simulink model "MyModel_Open_v1"  (R2018b)
settings: Solver=VariableStepAuto  StartTime=0.0  StopTime=10.0  RelTol=1e-3
InitFcn:
  | Udc1 = 100;
  | Udc2 = 100;
undefined symbols (not defined in the file): tpwm
libraries: powerlib x31, powerlib_meascontrol x28, powerlib_extras x5, simulink x2
(part 1 of 2)
settings Model: Creator=chenhao  LastModifiedBy=chenhao

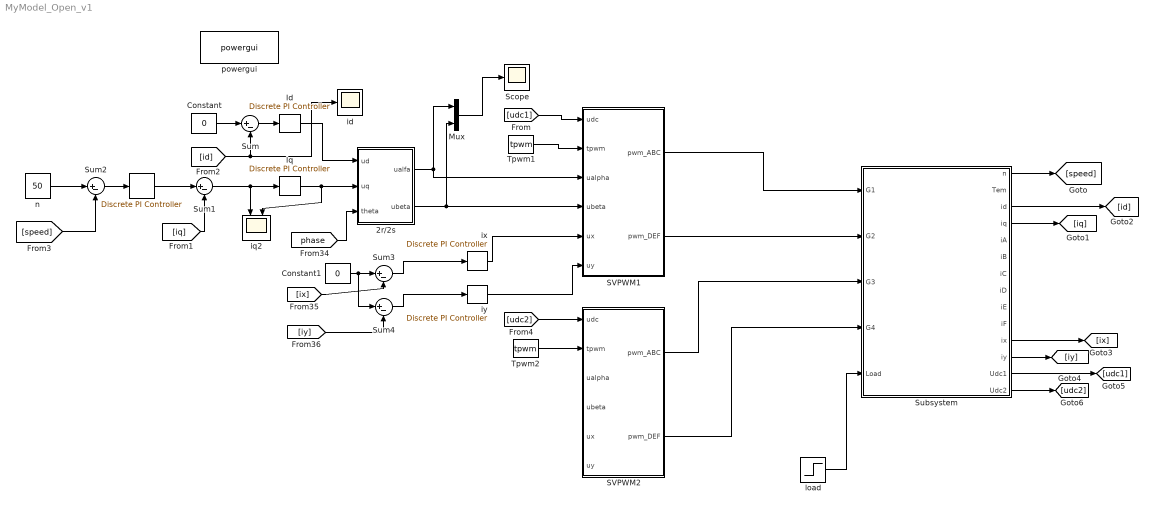
== system MyModel_Open_v1 ==
  "    " : powerlib_extras/Discrete  Control Blocks/Discrete PI Controller  Kp=1  Ki=80  Par_Limits=[50 -50]  Init=0  Ts=tpwm
  " Id" : powerlib_extras/Discrete  Control Blocks/Discrete PI Controller  Kp=3  Ki=120  Par_Limits=[300 -300]  Init=0  Ts=tpwm
  " Iq" : powerlib_extras/Discrete  Control Blocks/Discrete PI Controller  Kp=3  Ki=120  Par_Limits=[300 -300]  Init=0  Ts=tpwm
  " ix" : powerlib_extras/Discrete  Control Blocks/Discrete PI Controller  Kp=10  Ki=100  Par_Limits=[300 -300]  Init=0  Ts=tpwm
  " iy" : powerlib_extras/Discrete  Control Blocks/Discrete PI Controller  Kp=10  Ki=100  Par_Limits=[300 -300]  Init=0  Ts=tpwm
  2r/2s : Subsystem
  Constant : Constant  Value=0
  Constant1 : Constant  Value=0
  Mux : Mux  Inputs=2
  SVPWM1 : Subsystem
  SVPWM2 : Subsystem
  Scope : Scope
  Subsystem : Subsystem
  Sum{,1..4} (5 alike) : Sum  Inputs=|+-
  Tpwm1 : Constant  Value=tpwm
  Tpwm2 : Constant  Value=tpwm
  "id " : Scope
  iq2 : Scope  NumInputPorts=2
  load : Step  Time=0  After=15  SampleTime=0
  n : Constant  Value=50
  powergui : powerlib/powergui  Priority=1  SimulationMode=Discrete  SampleTime=5e-7  frequency=60  Iterations=50  frequencyindice=0  Pbase=100e6  ErrMax=1e-4  UnitsV=kV  UnitsW=MW  buscounter=0  FunctionMessages=off  echomessages=off  EnableUseOfTLC=off  CurrentSourceSwitches=off  DisableSnubberDevices=off  DisableRonSwitches=off  DisableVfSwitches=off  DisplayEquations=off  SolverType=Tustin  Interpol=off  ExternalGateDelay=off  methode=off  Ts=0  x0status=blocks  SPID=off  SwTol=0  HookPort=off  RestoreLinks=warning  ResistiveCurrentMeasurement=off  Frange=[0:2:500]  Ylog=off  Xlog=on  ShowGrid=off  save=off  variable=ZData  structure=Ia  ZoomFFT=on  StartTime=0.1  cycles=2  DisplayStyle=1  fundamental=2.5  FreqAxis=on  MaxFrequency=30  frequencyindicesteady=1  RmsSteady=1  display=off
  wires:
  2r/2s/2(ubeta) -> Mux/2, SVPWM1/4(ubeta)
  " ix"/1 -> SVPWM1/5(ux)
  Mux/1 -> Scope/1
  Tpwm1/1 -> SVPWM1/2(tpwm)
  load/1 -> Subsystem/5(Load)
  [iy] -> Sum4/2
  [iq] -> Sum1/2
  Sum3/1 -> " ix"/1
  [udc1] -> SVPWM1/1(udc)
  SVPWM1/1(pwm_ABC) -> Subsystem/1(G1)
  SVPWM1/2(pwm_DEF) -> Subsystem/2(G2)
  Sum2/1 -> "    "/1
  2r/2s/1(ualfa) -> Mux/1, SVPWM1/3(ualpha)
  Sum1/1 -> iq2/1, " Iq"/1
  [speed] -> Sum2/2
  Sum4/1 -> " iy"/1
  n/1 -> Sum2/1
  [ix] -> Sum3/2
  " Id"/1 -> 2r/2s/1(ud)
  [phase] -> 2r/2s/3(theta)
  " Iq"/1 -> iq2/2, 2r/2s/2(uq)
  Sum/1 -> " Id"/1
  Constant1/1 -> Sum4/1, Sum3/1
  "    "/1 -> Sum1/1
  " iy"/1 -> SVPWM1/6(uy)
  [id] -> "id "/1, Sum/2
  Constant/1 -> Sum/1
  Subsystem/1(n) -> [speed]
  Subsystem/4(iq) -> [iq]
  Subsystem/3(id) -> [id]
  Subsystem/11(ix) -> [ix]
  Subsystem/12(iy) -> [iy]
  Subsystem/13(Udc1) -> [udc1]
  Subsystem/14(Udc2) -> [udc2]
  [udc2] -> SVPWM2/1(udc)
  Tpwm2/1 -> SVPWM2/2(tpwm)
  SVPWM2/1(pwm_ABC) -> Subsystem/3(G3)
  SVPWM2/2(pwm_DEF) -> Subsystem/4(G4)

== system MyModel_Open_v1/2r//2s ==
  ud : Inport
  uq : Inport  Port=2
  theta : Inport  Port=3
  Fcn : Fcn  Expr=u(1)*cos(u(3))-u(2)*sin(u(3))
  Fcn1 : Fcn  Expr=u(1)*sin(u(3))+u(2)*cos(u(3))
  Mux1 : Mux  Inputs=3
  ualfa : Outport
  ubeta : Outport  Port=2
  wires:
  theta/1 -> Mux1/3
  uq/1 -> Mux1/2
  ud/1 -> Mux1/1
  Fcn1/1 -> ubeta/1
  Fcn/1 -> ualfa/1
  Mux1/1 -> Fcn1/1, Fcn/1

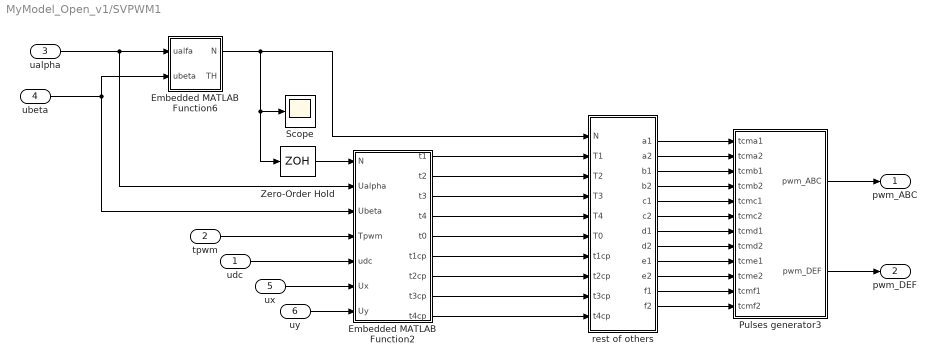
== system MyModel_Open_v1/SVPWM1 ==
  udc : Inport
  tpwm : Inport  Port=2
  ualpha : Inport  Port=3
  ubeta : Inport  Port=4
  ux : Inport  Port=5
  uy : Inport  Port=6
  Embedded MATLAB Function2 : MATLAB Function  TreatAsAtomicUnit=on
  Embedded MATLAB Function6 : MATLAB Function  TreatAsAtomicUnit=on
  Pulses generator3 : Subsystem
  Scope : Scope
  Zero-Order Hold : ZeroOrderHold  SampleTime=1e-4
  rest of others : MATLAB Function  TreatAsAtomicUnit=on
  pwm_ABC : Outport
  pwm_DEF : Outport  Port=2
  wires:
  udc/1 -> Embedded MATLAB Function2/5(udc)
  Embedded MATLAB Function2/4(t4) -> rest of others/5(T4)
  Embedded MATLAB Function2/1(t1) -> rest of others/2(T1)
  Pulses generator3/1(pwm_ABC) -> pwm_ABC/1
  Pulses generator3/2(pwm_DEF) -> pwm_DEF/1
  rest of others/12(f2) -> Pulses generator3/12(tcmf2)
  rest of others/11(f1) -> Pulses generator3/11(tcmf1)
  rest of others/10(e2) -> Pulses generator3/10(tcme2)
  rest of others/9(e1) -> Pulses generator3/9(tcme1)
  rest of others/8(d2) -> Pulses generator3/8(tcmd2)
  rest of others/7(d1) -> Pulses generator3/7(tcmd1)
  rest of others/6(c2) -> Pulses generator3/6(tcmc2)
  rest of others/5(c1) -> Pulses generator3/5(tcmc1)
  rest of others/4(b2) -> Pulses generator3/4(tcmb2)
  rest of others/3(b1) -> Pulses generator3/3(tcmb1)
  rest of others/2(a2) -> Pulses generator3/2(tcma2)
  rest of others/1(a1) -> Pulses generator3/1(tcma1)
  Embedded MATLAB Function2/2(t2) -> rest of others/3(T2)
  tpwm/1 -> Embedded MATLAB Function2/4(Tpwm)
  Embedded MATLAB Function2/5(t0) -> rest of others/6(T0)
  ualpha/1 -> Embedded MATLAB Function2/2(Ualpha), Embedded MATLAB Function6/1(ualfa)
  ubeta/1 -> Embedded MATLAB Function6/2(ubeta), Embedded MATLAB Function2/3(Ubeta)
  ux/1 -> Embedded MATLAB Function2/6(Ux)
  uy/1 -> Embedded MATLAB Function2/7(Uy)
  Embedded MATLAB Function2/3(t3) -> rest of others/4(T3)
  Zero-Order Hold/1 -> Embedded MATLAB Function2/1(N)
  Embedded MATLAB Function6/1(N) -> rest of others/1(N), Scope/1, Zero-Order Hold/1
  Embedded MATLAB Function2/9(t4cp) -> rest of others/10(t4cp)
  Embedded MATLAB Function2/8(t3cp) -> rest of others/9(t3cp)
  Embedded MATLAB Function2/7(t2cp) -> rest of others/8(t2cp)
  Embedded MATLAB Function2/6(t1cp) -> rest of others/7(t1cp)

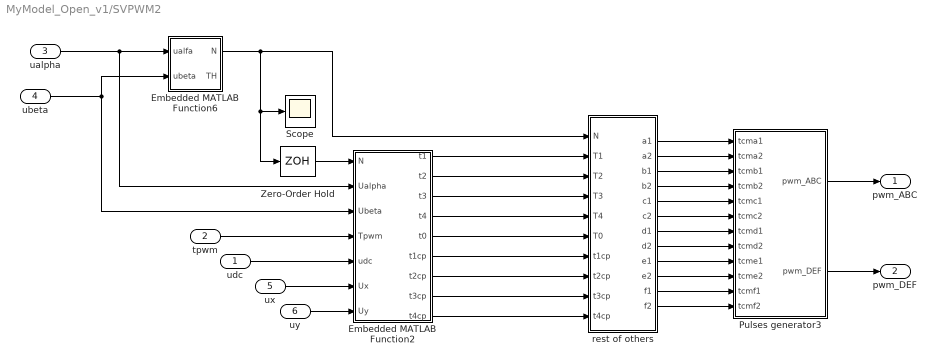
== system MyModel_Open_v1/SVPWM2 ==
  udc : Inport
  tpwm : Inport  Port=2
  ualpha : Inport  Port=3
  ubeta : Inport  Port=4
  ux : Inport  Port=5
  uy : Inport  Port=6
  Embedded MATLAB Function2 : MATLAB Function  TreatAsAtomicUnit=on
  Embedded MATLAB Function6 : MATLAB Function  TreatAsAtomicUnit=on
  Pulses generator3 : Subsystem
  Scope : Scope
  Zero-Order Hold : ZeroOrderHold  SampleTime=1e-4
  rest of others : MATLAB Function  TreatAsAtomicUnit=on
  pwm_ABC : Outport
  pwm_DEF : Outport  Port=2
  wires:
  Embedded MATLAB Function2/6(t1cp) -> rest of others/7(t1cp)
  Embedded MATLAB Function2/7(t2cp) -> rest of others/8(t2cp)
  Embedded MATLAB Function2/8(t3cp) -> rest of others/9(t3cp)
  Embedded MATLAB Function2/9(t4cp) -> rest of others/10(t4cp)
  Embedded MATLAB Function6/1(N) -> Zero-Order Hold/1, Scope/1, rest of others/1(N)
  Zero-Order Hold/1 -> Embedded MATLAB Function2/1(N)
  Embedded MATLAB Function2/3(t3) -> rest of others/4(T3)
  uy/1 -> Embedded MATLAB Function2/7(Uy)
  ux/1 -> Embedded MATLAB Function2/6(Ux)
  ubeta/1 -> Embedded MATLAB Function2/3(Ubeta), Embedded MATLAB Function6/2(ubeta)
  ualpha/1 -> Embedded MATLAB Function6/1(ualfa), Embedded MATLAB Function2/2(Ualpha)
  Embedded MATLAB Function2/5(t0) -> rest of others/6(T0)
  tpwm/1 -> Embedded MATLAB Function2/4(Tpwm)
  Embedded MATLAB Function2/2(t2) -> rest of others/3(T2)
  rest of others/1(a1) -> Pulses generator3/1(tcma1)
  rest of others/2(a2) -> Pulses generator3/2(tcma2)
  rest of others/3(b1) -> Pulses generator3/3(tcmb1)
  rest of others/4(b2) -> Pulses generator3/4(tcmb2)
  rest of others/5(c1) -> Pulses generator3/5(tcmc1)
  rest of others/6(c2) -> Pulses generator3/6(tcmc2)
  rest of others/7(d1) -> Pulses generator3/7(tcmd1)
  rest of others/8(d2) -> Pulses generator3/8(tcmd2)
  rest of others/9(e1) -> Pulses generator3/9(tcme1)
  rest of others/10(e2) -> Pulses generator3/10(tcme2)
  rest of others/11(f1) -> Pulses generator3/11(tcmf1)
  rest of others/12(f2) -> Pulses generator3/12(tcmf2)
  Pulses generator3/2(pwm_DEF) -> pwm_DEF/1
  Pulses generator3/1(pwm_ABC) -> pwm_ABC/1
  Embedded MATLAB Function2/1(t1) -> rest of others/2(T1)
  Embedded MATLAB Function2/4(t4) -> rest of others/5(T4)
  udc/1 -> Embedded MATLAB Function2/5(udc)

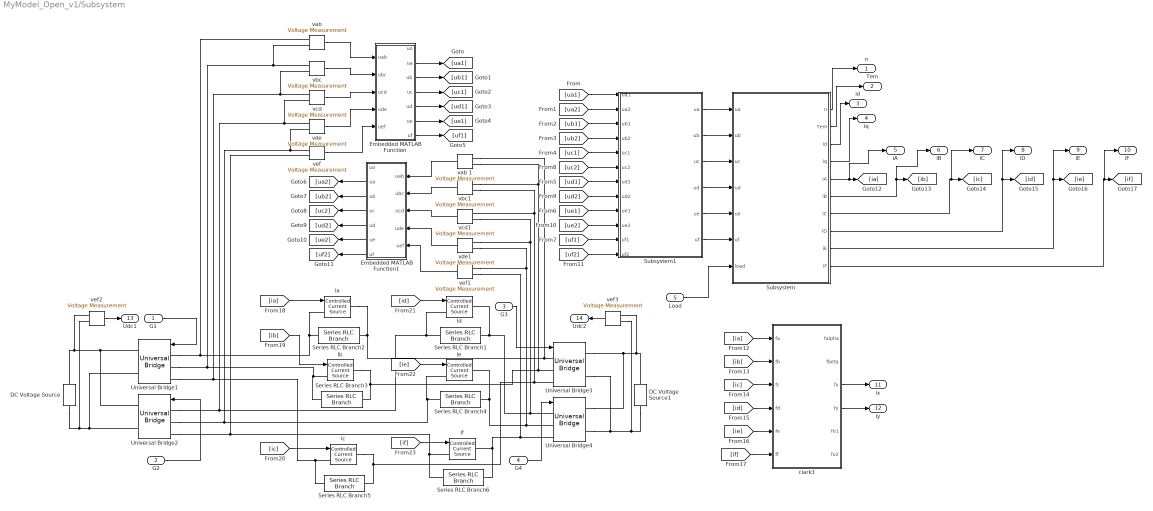
== system MyModel_Open_v1/Subsystem ==
  G1 : Inport
  G2 : Inport  Port=2
  G3 : Inport  Port=3
  G4 : Inport  Port=4
  Load : Inport  Port=5
  DC Voltage Source : powerlib/Electrical Sources/DC Voltage Source  Amplitude=Udc1  Measurements=Voltage
  DC Voltage Source1 : powerlib/Electrical Sources/DC Voltage Source  Amplitude=Udc2  Measurements=Voltage
  Embedded MATLAB Function : MATLAB Function  TreatAsAtomicUnit=on
  Embedded MATLAB Function1 : MATLAB Function  TreatAsAtomicUnit=on
  Id : powerlib/Electrical Sources/Controlled Current Source  Initialize=on  Source_Type=AC  Amplitude=0  Phase=0  Frequency=0  Measurements=None
  Series RLC Branch{1..6} (6 alike) : powerlib/Elements/Series RLC Branch  LConnTagsString=__new0  RConnTagsString=__new0  BranchType=R  Resistance=10e10  Inductance=10e-7  SetiL0=off  InitialCurrent=0  Capacitance=1e-6  Setx0=off  InitialVoltage=0  Measurements=None
  Subsystem : Subsystem
  Subsystem1 : Subsystem
  Universal Bridge{1..4} (4 alike) : powerlib/Power Electronics/Universal Bridge  Arms=3  SnubberResistance=1e5  SnubberCapacitance=inf  Device=IGBT / Diodes  Ron=1e-3  Lon=0  ForwardVoltages="[  0  0  ]"  ForwardVoltage=0  GTOparameters=[ 10e-6 , 20e-6 ]  IGBTparameters=[ 0 , 0 ]  Measurements=None  Measurements_2=None  converterType=Rectifier
  clark1 : MATLAB Function  TreatAsAtomicUnit=on
  ia : powerlib/Electrical Sources/Controlled Current Source  Initialize=on  Source_Type=AC  Amplitude=0  Phase=0  Frequency=0  Measurements=None
  ib : powerlib/Electrical Sources/Controlled Current Source  Initialize=on  Source_Type=AC  Amplitude=0  Phase=0  Frequency=0  Measurements=None
  ic : powerlib/Electrical Sources/Controlled Current Source  Initialize=on  Source_Type=AC  Amplitude=0  Phase=0  Frequency=0  Measurements=None
  ie : powerlib/Electrical Sources/Controlled Current Source  Initialize=on  Source_Type=AC  Amplitude=0  Phase=0  Frequency=0  Measurements=None
  if : powerlib/Electrical Sources/Controlled Current Source  Initialize=on  Source_Type=AC  Amplitude=0  Phase=0  Frequency=0  Measurements=None
  "vab " : powerlib/Measurements/Voltage Measurement  PhasorSimulation=off  OutputType=Complex  PSBequivalent=0
  vab 1 : powerlib/Measurements/Voltage Measurement  PhasorSimulation=off  OutputType=Complex  PSBequivalent=0
  vbc : powerlib/Measurements/Voltage Measurement  PhasorSimulation=off  OutputType=Complex  PSBequivalent=0
  vbc1 : powerlib/Measurements/Voltage Measurement  PhasorSimulation=off  OutputType=Complex  PSBequivalent=0
  vcd : powerlib/Measurements/Voltage Measurement  PhasorSimulation=off  OutputType=Complex  PSBequivalent=0
  vcd1 : powerlib/Measurements/Voltage Measurement  PhasorSimulation=off  OutputType=Complex  PSBequivalent=0
  vde : powerlib/Measurements/Voltage Measurement  PhasorSimulation=off  OutputType=Complex  PSBequivalent=0
  vde1 : powerlib/Measurements/Voltage Measurement  PhasorSimulation=off  OutputType=Complex  PSBequivalent=0
  vef{,1..3} (4 alike) : powerlib/Measurements/Voltage Measurement  PhasorSimulation=off  OutputType=Complex  PSBequivalent=0
  n : Outport
  Tem : Outport  Port=2
  id : Outport  Port=3
  iq : Outport  Port=4
  iA : Outport  Port=5
  iB : Outport  Port=6
  iC : Outport  Port=7
  iD : Outport  Port=8
  iE : Outport  Port=9
  iF : Outport  Port=10
  ix : Outport  Port=11
  iy : Outport  Port=12
  Udc1 : Outport  Port=13
  Udc2 : Outport  Port=14
  wires:
  G1/1 -> Universal Bridge1/1
  G2/1 -> Universal Bridge2/1
  G3/1 -> Universal Bridge3/1
  G4/1 -> Universal Bridge4/1
  vef/1 -> Embedded MATLAB Function/5(uef)
  vde/1 -> Embedded MATLAB Function/4(ude)
  "vab "/1 -> Embedded MATLAB Function/1(uab)
  vcd/1 -> Embedded MATLAB Function/3(ucd)
  vbc/1 -> Embedded MATLAB Function/2(ubc)
  Embedded MATLAB Function/2(ua) -> [ua1]
  Embedded MATLAB Function/3(ub) -> [ub1]
  Embedded MATLAB Function/4(uc) -> [uc1]
  Embedded MATLAB Function/5(ud) -> [ud1]
  Embedded MATLAB Function/6(ue) -> [ue1]
  Embedded MATLAB Function/7(uf) -> [uf1]
  Embedded MATLAB Function1/2(ua) -> [ua2]
  Embedded MATLAB Function1/3(ub) -> [ub2]
  Embedded MATLAB Function1/4(uc) -> [uc2]
  Embedded MATLAB Function1/5(ud) -> [ud2]
  Embedded MATLAB Function1/6(ue) -> [ue2]
  Embedded MATLAB Function1/7(uf) -> [uf2]
  vab 1/1 -> Embedded MATLAB Function1/1(uab)
  vbc1/1 -> Embedded MATLAB Function1/2(ubc)
  vcd1/1 -> Embedded MATLAB Function1/3(ucd)
  vde1/1 -> Embedded MATLAB Function1/4(ude)
  vef1/1 -> Embedded MATLAB Function1/5(uef)
  [ua1] -> Subsystem1/1(ua1)
  [ua2] -> Subsystem1/2(ua2)
  [ub1] -> Subsystem1/3(ub1)
  [ub2] -> Subsystem1/4(ub2)
  [uc1] -> Subsystem1/5(uc1)
  [uc2] -> Subsystem1/6(uc2)
  [ud1] -> Subsystem1/7(ud1)
  [ud2] -> Subsystem1/8(ud2)
  [ue1] -> Subsystem1/9(ue1)
  [ue2] -> Subsystem1/10(ue2)
  [uf1] -> Subsystem1/11(uf1)
  [uf2] -> Subsystem1/12(uf2)
  Subsystem1/1(ua) -> Subsystem/1(ua)
  Subsystem1/2(ub) -> Subsystem/2(ub)
  Subsystem1/3(uc) -> Subsystem/3(uc)
  Subsystem1/4(ud) -> Subsystem/4(ud)
  Subsystem1/5(ue) -> Subsystem/5(ue)
  Subsystem1/6(uf) -> Subsystem/6(uf)
  Load/1 -> Subsystem/7(load)
  Subsystem/1(n) -> n/1
  Subsystem/2(Tem) -> Tem/1
  Subsystem/3(id) -> id/1
  Subsystem/4(iq) -> iq/1
  Subsystem/5(iA) -> iA/1, [ia]
  Subsystem/6(iB) -> iB/1, [ib]
  Subsystem/7(iC) -> iC/1, [ic]
  Subsystem/8(iD) -> iD/1, [id]
  Subsystem/9(iE) -> iE/1, [ie]
  Subsystem/10(iF) -> iF/1, [if]
  [ia] -> clark1/1(fa)
  [ib] -> clark1/2(fb)
  [ic] -> clark1/3(fc)
  [id] -> clark1/4(fd)
  [ie] -> clark1/5(fe)
  [if] -> clark1/6(ff)
  clark1/3(fx) -> ix/1
  clark1/4(fy) -> iy/1
  vef2/1 -> Udc1/1
  vef3/1 -> Udc2/1
  [ia] -> ia/1
  [ib] -> ib/1
  [ic] -> ic/1
  [id] -> Id/1
  [ie] -> ie/1
  [if] -> if/1
  connections:
  Series RLC Branch1/RConn1 -- Universal Bridge4/LConn1 -- vde1/LConn1 -- vcd1/LConn2 -- Id/RConn1
  Series RLC Branch1/LConn1 -- vde/LConn1 -- vcd/LConn2 -- Universal Bridge2/LConn1 -- Id/LConn1
  Series RLC Branch4/LConn1 -- vef/LConn1 -- vde/LConn2 -- Universal Bridge2/LConn2 -- ie/LConn1
  Series RLC Branch6/LConn1 -- vef/LConn2 -- Universal Bridge2/LConn3 -- if/LConn1
  Series RLC Branch6/RConn1 -- Universal Bridge4/LConn3 -- vef1/LConn2 -- if/RConn1
  Universal Bridge1/RConn2 -- vef2/LConn2 -- DC Voltage Source/LConn1 -- Universal Bridge2/RConn2
  DC Voltage Source/RConn1 -- vef2/LConn1 -- Universal Bridge2/RConn1 -- Universal Bridge1/RConn1
  ia/LConn1 -- "vab "/LConn1 -- Universal Bridge1/LConn1 -- Series RLC Branch2/LConn1
  ia/RConn1 -- vab 1/LConn1 -- Universal Bridge3/LConn1 -- Series RLC Branch2/RConn1
  ib/LConn1 -- vbc/LConn1 -- "vab "/LConn2 -- Universal Bridge1/LConn2 -- Series RLC Branch3/LConn1
  ib/RConn1 -- Series RLC Branch3/RConn1 -- vbc1/LConn1 -- vab 1/LConn2 -- Universal Bridge3/LConn2
  ic/LConn1 -- vcd/LConn1 -- vbc/LConn2 -- Universal Bridge1/LConn3 -- Series RLC Branch5/LConn1
  vbc1/LConn2 -- ic/RConn1 -- Series RLC Branch5/RConn1 -- Universal Bridge3/LConn3 -- vcd1/LConn1
  Universal Bridge3/RConn1 -- vef3/LConn1 -- DC Voltage Source1/RConn1 -- Universal Bridge4/RConn1
  Universal Bridge3/RConn2 -- vef3/LConn2 -- DC Voltage Source1/LConn1 -- Universal Bridge4/RConn2
  vef1/LConn1 -- Series RLC Branch4/RConn1 -- ie/RConn1 -- Universal Bridge4/LConn2 -- vde1/LConn2

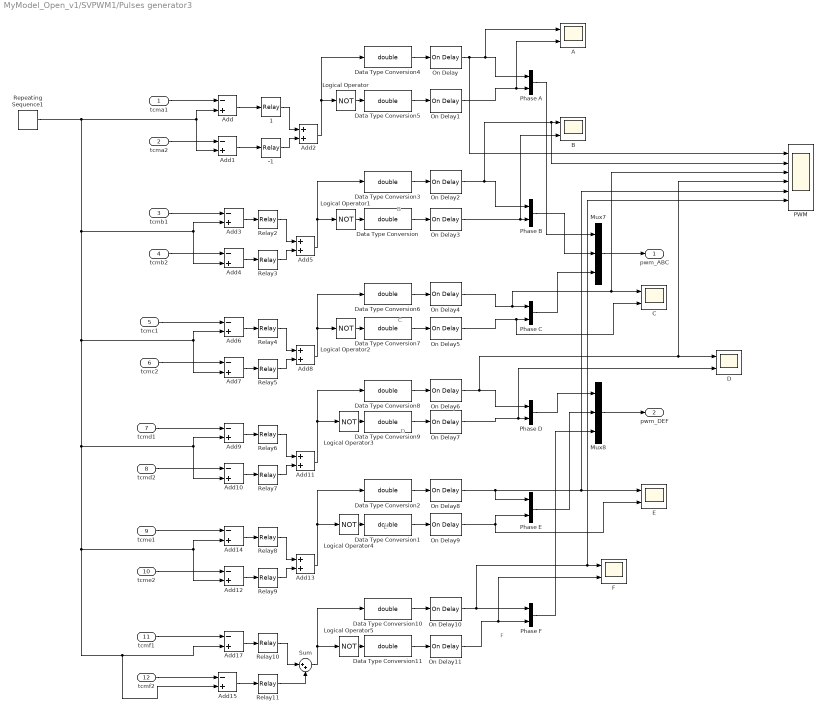
== system MyModel_Open_v1/SVPWM1/Pulses generator3 ==
  note: B
  note: C
  note: D
  note: E
  note: F
  tcma1 : Inport
  tcma2 : Inport  Port=2
  tcmb1 : Inport  Port=3
  tcmb2 : Inport  Port=4
  tcmc1 : Inport  Port=5
  tcmc2 : Inport  Port=6
  tcmd1 : Inport  Port=7
  tcmd2 : Inport  Port=8
  tcme1 : Inport  Port=9
  tcme2 : Inport  Port=10
  tcmf1 : Inport  Port=11
  tcmf2 : Inport  Port=12
  -1 : Relay  OnOutputValue=-1
  1 : Relay
  A : Scope  NumInputPorts=2
  Add{,1,3..4,6..7,9..10,12,14..15,17} (12 alike) : Sum  Inputs=-+
  Add{2,5,8,11,13} (5 alike) : Sum
  B : Scope  NumInputPorts=2
  C : Scope  NumInputPorts=2
  D : Scope  NumInputPorts=2
  Data Type Conversion{,1..11} (12 alike) : DataTypeConversion  OutDataTypeStr=double
  E : Scope  NumInputPorts=2
  F : Scope  NumInputPorts=2
  Logical Operator{,1..5} (6 alike) : Logic  Operator=NOT  AllPortsSameDT=off  OutDataTypeStr=boolean
  Mux7 : Mux  Inputs=3
  Mux8 : Mux  Inputs=3
  On Delay{,1..11} (12 alike) : powerlib_meascontrol/Logic/On Delay  DelayType=On delay  delay=Td  ic=0  Ts=0
      settings: SourceProductName=Simscape Power Systems
  PWM : Scope  NumInputPorts=6
  Phase A : Mux  Inputs=2
  Phase B : Mux  Inputs=2
  Phase C : Mux  Inputs=2
  Phase D : Mux  Inputs=2
  Phase E : Mux  Inputs=2
  Phase F : Mux  Inputs=2
  Relay{2,4,6,8,10} (5 alike) : Relay
  Relay{3,5,7,9,11} (5 alike) : Relay  OnOutputValue=-1
  Repeating Sequence1 : simulink/Sources/Repeating Sequence  rep_seq_t=[0 tpwm]  rep_seq_y=[0 tpwm]
  Sum : Sum  Inputs=|++
  pwm_ABC : Outport
  pwm_DEF : Outport  Port=2
  wires:
  On Delay11/1 -> F/2, Phase F/2
  Data Type Conversion11/1 -> On Delay11/1
  On Delay10/1 -> PWM/6, F/1, Phase F/1
  Data Type Conversion10/1 -> On Delay10/1
  On Delay9/1 -> E/2, Phase E/2
  Data Type Conversion1/1 -> On Delay9/1
  On Delay8/1 -> Phase E/1, PWM/5, E/1
  Data Type Conversion2/1 -> On Delay8/1
  On Delay7/1 -> D/2, Phase D/2
  Data Type Conversion9/1 -> On Delay7/1
  On Delay6/1 -> PWM/4, D/1, Phase D/1
  Data Type Conversion8/1 -> On Delay6/1
  On Delay5/1 -> C/2, Phase C/2
  Data Type Conversion7/1 -> On Delay5/1
  On Delay4/1 -> PWM/3, C/1, Phase C/1
  Data Type Conversion6/1 -> On Delay4/1
  On Delay2/1 -> PWM/2, B/1, Phase B/1
  On Delay3/1 -> B/2, Phase B/2
  Data Type Conversion/1 -> On Delay3/1
  Data Type Conversion3/1 -> On Delay2/1
  On Delay1/1 -> A/2, Phase A/2
  Data Type Conversion5/1 -> On Delay1/1
  On Delay/1 -> A/1, Phase A/1, PWM/1
  Data Type Conversion4/1 -> On Delay/1
  Logical Operator3/1 -> Data Type Conversion9/1
  Logical Operator2/1 -> Data Type Conversion7/1
  Logical Operator/1 -> Data Type Conversion5/1
  Logical Operator1/1 -> Data Type Conversion/1
  Logical Operator4/1 -> Data Type Conversion1/1
  Add5/1 -> Logical Operator1/1, Data Type Conversion3/1
  Add2/1 -> Logical Operator/1, Data Type Conversion4/1
  Mux8/1 -> pwm_DEF/1
  Mux7/1 -> pwm_ABC/1
  Sum/1 -> Logical Operator5/1, Data Type Conversion10/1
  Add13/1 -> Logical Operator4/1, Data Type Conversion2/1
  Add11/1 -> Logical Operator3/1, Data Type Conversion8/1
  Add8/1 -> Logical Operator2/1, Data Type Conversion6/1
  Logical Operator5/1 -> Data Type Conversion11/1
  tcmf2/1 -> Add15/1
  Relay11/1 -> Sum/2
  Relay10/1 -> Sum/1
  Add17/1 -> Relay10/1
  tcmf1/1 -> Add17/1
  tcme2/1 -> Add12/1
  Relay9/1 -> Add13/2
  Relay8/1 -> Add13/1
  Add12/1 -> Relay9/1
  Add14/1 -> Relay8/1
  tcme1/1 -> Add14/1
  tcmd2/1 -> Add10/1
  Relay7/1 -> Add11/2
  Relay6/1 -> Add11/1
  Add10/1 -> Relay7/1
  Add9/1 -> Relay6/1
  tcmd1/1 -> Add9/1
  tcmc2/1 -> Add7/1
  Relay5/1 -> Add8/2
  Relay4/1 -> Add8/1
  Add7/1 -> Relay5/1
  Add6/1 -> Relay4/1
  tcmb2/1 -> Add4/1
  Relay3/1 -> Add5/2
  Relay2/1 -> Add5/1
  Add4/1 -> Relay3/1
  Add3/1 -> Relay2/1
  tcma1/1 -> Add/1
  -1/1 -> Add2/2
  1/1 -> Add2/1
  Add1/1 -> -1/1
  Add/1 -> 1/1
  Repeating Sequence1/1 -> Add15/2, Add17/2, Add12/2, Add14/2, Add9/2, Add10/2, Add7/2, Add6/2, Add3/2, Add4/2, Add1/2, Add/2
  tcma2/1 -> Add1/1
  tcmb1/1 -> Add3/1
  tcmc1/1 -> Add6/1
  Add15/1 -> Relay11/1
  Phase A/1 -> Mux7/1
  Phase B/1 -> Mux7/2
  Phase C/1 -> Mux7/3
  Phase D/1 -> Mux8/1
  Phase E/1 -> Mux8/2
  Phase F/1 -> Mux8/3

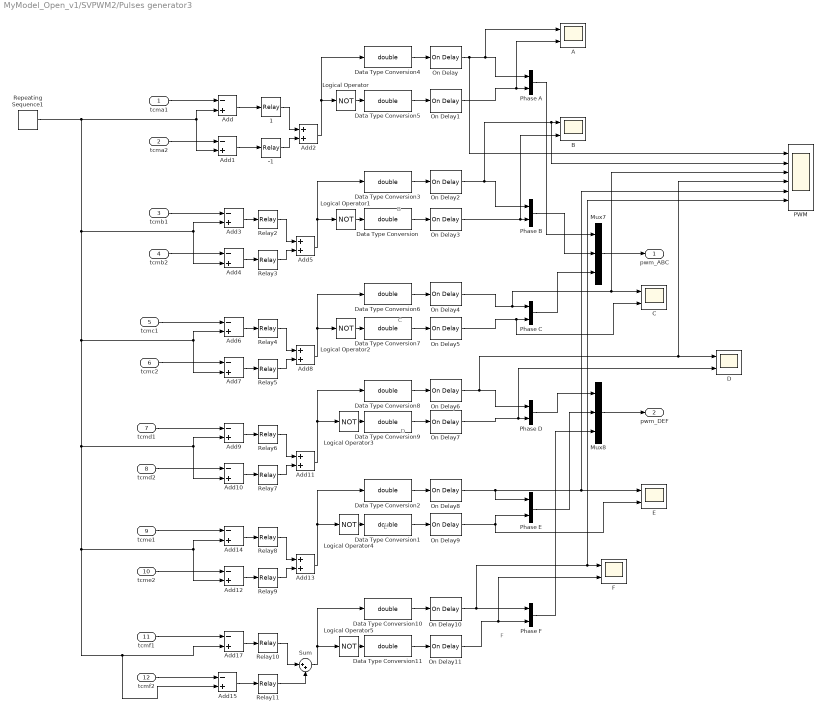
== system MyModel_Open_v1/SVPWM2/Pulses generator3 ==
  note: F
  note: E
  note: D
  note: C
  note: B
  tcma1 : Inport
  tcma2 : Inport  Port=2
  tcmb1 : Inport  Port=3
  tcmb2 : Inport  Port=4
  tcmc1 : Inport  Port=5
  tcmc2 : Inport  Port=6
  tcmd1 : Inport  Port=7
  tcmd2 : Inport  Port=8
  tcme1 : Inport  Port=9
  tcme2 : Inport  Port=10
  tcmf1 : Inport  Port=11
  tcmf2 : Inport  Port=12
  -1 : Relay  OnOutputValue=-1
  1 : Relay
  A : Scope  NumInputPorts=2
  Add{,1,3..4,6..7,9..10,12,14..15,17} (12 alike) : Sum  Inputs=-+
  Add{2,5,8,11,13} (5 alike) : Sum
  B : Scope  NumInputPorts=2
  C : Scope  NumInputPorts=2
  D : Scope  NumInputPorts=2
  Data Type Conversion{,1..11} (12 alike) : DataTypeConversion  OutDataTypeStr=double
  E : Scope  NumInputPorts=2
  F : Scope  NumInputPorts=2
  Logical Operator{,1..5} (6 alike) : Logic  Operator=NOT  AllPortsSameDT=off  OutDataTypeStr=boolean
  Mux7 : Mux  Inputs=3
  Mux8 : Mux  Inputs=3
  On Delay{,1..11} (12 alike) : powerlib_meascontrol/Logic/On Delay  DelayType=On delay  delay=Td  ic=0  Ts=0
      settings: SourceProductName=Simscape Power Systems
  PWM : Scope  NumInputPorts=6
  Phase A : Mux  Inputs=2
  Phase B : Mux  Inputs=2
  Phase C : Mux  Inputs=2
  Phase D : Mux  Inputs=2
  Phase E : Mux  Inputs=2
  Phase F : Mux  Inputs=2
  Relay{2,4,6,8,10} (5 alike) : Relay
  Relay{3,5,7,9,11} (5 alike) : Relay  OnOutputValue=-1
  Repeating Sequence1 : simulink/Sources/Repeating Sequence  rep_seq_t=[0 tpwm]  rep_seq_y=[0 tpwm]
  Sum : Sum  Inputs=|++
  pwm_ABC : Outport
  pwm_DEF : Outport  Port=2
  wires:
  Phase F/1 -> Mux8/3
  Phase E/1 -> Mux8/2
  Phase D/1 -> Mux8/1
  Phase C/1 -> Mux7/3
  Phase B/1 -> Mux7/2
  Phase A/1 -> Mux7/1
  Add15/1 -> Relay11/1
  tcmc1/1 -> Add6/1
  tcmb1/1 -> Add3/1
  tcma2/1 -> Add1/1
  Repeating Sequence1/1 -> Add/2, Add1/2, Add4/2, Add3/2, Add6/2, Add7/2, Add10/2, Add9/2, Add14/2, Add12/2, Add17/2, Add15/2
  Add/1 -> 1/1
  Add1/1 -> -1/1
  1/1 -> Add2/1
  -1/1 -> Add2/2
  tcma1/1 -> Add/1
  Add3/1 -> Relay2/1
  Add4/1 -> Relay3/1
  Relay2/1 -> Add5/1
  Relay3/1 -> Add5/2
  tcmb2/1 -> Add4/1
  Add6/1 -> Relay4/1
  Add7/1 -> Relay5/1
  Relay4/1 -> Add8/1
  Relay5/1 -> Add8/2
  tcmc2/1 -> Add7/1
  tcmd1/1 -> Add9/1
  Add9/1 -> Relay6/1
  Add10/1 -> Relay7/1
  Relay6/1 -> Add11/1
  Relay7/1 -> Add11/2
  tcmd2/1 -> Add10/1
  tcme1/1 -> Add14/1
  Add14/1 -> Relay8/1
  Add12/1 -> Relay9/1
  Relay8/1 -> Add13/1
  Relay9/1 -> Add13/2
  tcme2/1 -> Add12/1
  tcmf1/1 -> Add17/1
  Add17/1 -> Relay10/1
  Relay10/1 -> Sum/1
  Relay11/1 -> Sum/2
  tcmf2/1 -> Add15/1
  Logical Operator5/1 -> Data Type Conversion11/1
  Add8/1 -> Data Type Conversion6/1, Logical Operator2/1
  Add11/1 -> Data Type Conversion8/1, Logical Operator3/1
  Add13/1 -> Data Type Conversion2/1, Logical Operator4/1
  Sum/1 -> Data Type Conversion10/1, Logical Operator5/1
  Mux7/1 -> pwm_ABC/1
  Mux8/1 -> pwm_DEF/1
  Add2/1 -> Data Type Conversion4/1, Logical Operator/1
  Add5/1 -> Data Type Conversion3/1, Logical Operator1/1
  Logical Operator4/1 -> Data Type Conversion1/1
  Logical Operator1/1 -> Data Type Conversion/1
  Logical Operator/1 -> Data Type Conversion5/1
  Logical Operator2/1 -> Data Type Conversion7/1
  Logical Operator3/1 -> Data Type Conversion9/1
  Data Type Conversion4/1 -> On Delay/1
  On Delay/1 -> PWM/1, Phase A/1, A/1
  Data Type Conversion5/1 -> On Delay1/1
  On Delay1/1 -> Phase A/2, A/2
  Data Type Conversion3/1 -> On Delay2/1
  Data Type Conversion/1 -> On Delay3/1
  On Delay3/1 -> Phase B/2, B/2
  On Delay2/1 -> Phase B/1, B/1, PWM/2
  Data Type Conversion6/1 -> On Delay4/1
  On Delay4/1 -> Phase C/1, C/1, PWM/3
  Data Type Conversion7/1 -> On Delay5/1
  On Delay5/1 -> Phase C/2, C/2
  Data Type Conversion8/1 -> On Delay6/1
  On Delay6/1 -> Phase D/1, D/1, PWM/4
  Data Type Conversion9/1 -> On Delay7/1
  On Delay7/1 -> Phase D/2, D/2
  Data Type Conversion2/1 -> On Delay8/1
  On Delay8/1 -> E/1, PWM/5, Phase E/1
  Data Type Conversion1/1 -> On Delay9/1
  On Delay9/1 -> Phase E/2, E/2
  Data Type Conversion10/1 -> On Delay10/1
  On Delay10/1 -> Phase F/1, F/1, PWM/6
  Data Type Conversion11/1 -> On Delay11/1
  On Delay11/1 -> Phase F/2, F/2

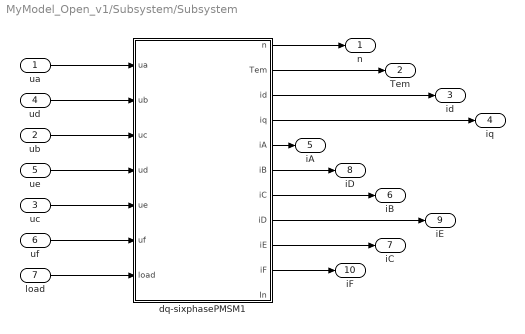
== system MyModel_Open_v1/Subsystem/Subsystem ==
  ua : Inport
  ub : Inport  Port=2
  uc : Inport  Port=3
  ud : Inport  Port=4
  ue : Inport  Port=5
  uf : Inport  Port=6
  load : Inport  Port=7
  dq-sixphasePMSM1 : Subsystem  mask{R=0.099, Ld=2.463342136542000e-03, Lq=2.473254136542000e-03, Lf=1.520747e-3, psi=0.0592, p=5, J=0.00174}
      mask prompts: R "Resistance (Om)"; Ld "d-inductance (H)"; Lq "q-inductance (H)"; Lf "Leak inductance (H)"; psi "flux (Wb)"; p "pole pairs"; J "inertia (kg*m^2)"
  n : Outport
  Tem : Outport  Port=2
  id : Outport  Port=3
  iq : Outport  Port=4
  iA : Outport  Port=5
  iB : Outport  Port=6
  iC : Outport  Port=7
  iD : Outport  Port=8
  iE : Outport  Port=9
  iF : Outport  Port=10
  wires:
  dq-sixphasePMSM1/10(iF) -> iF/1
  dq-sixphasePMSM1/4(iq) -> iq/1
  ue/1 -> dq-sixphasePMSM1/4(ud)
  dq-sixphasePMSM1/8(iD) -> iE/1
  uf/1 -> dq-sixphasePMSM1/6(uf)
  dq-sixphasePMSM1/7(iC) -> iB/1
  dq-sixphasePMSM1/5(iA) -> iA/1
  dq-sixphasePMSM1/2(Tem) -> Tem/1
  ua/1 -> dq-sixphasePMSM1/1(ua)
  dq-sixphasePMSM1/3(id) -> id/1
  ud/1 -> dq-sixphasePMSM1/2(ub)
  dq-sixphasePMSM1/9(iE) -> iC/1
  dq-sixphasePMSM1/1(n) -> n/1
  load/1 -> dq-sixphasePMSM1/7(load)
  uc/1 -> dq-sixphasePMSM1/5(ue)
  dq-sixphasePMSM1/6(iB) -> iD/1
  ub/1 -> dq-sixphasePMSM1/3(uc)

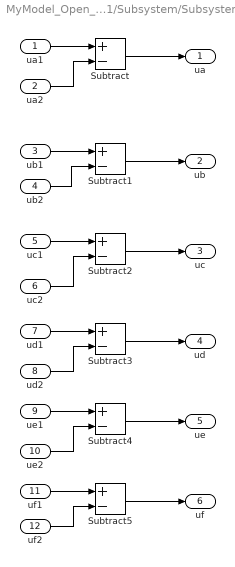
== system MyModel_Open_v1/Subsystem/Subsystem1 ==
  ua1 : Inport
  ua2 : Inport  Port=2
  ub1 : Inport  Port=3
  ub2 : Inport  Port=4
  uc1 : Inport  Port=5
  uc2 : Inport  Port=6
  ud1 : Inport  Port=7
  ud2 : Inport  Port=8
  ue1 : Inport  Port=9
  ue2 : Inport  Port=10
  uf1 : Inport  Port=11
  uf2 : Inport  Port=12
  Subtract{,1..5} (6 alike) : Sum  Inputs=+-
  ua : Outport
  ub : Outport  Port=2
  uc : Outport  Port=3
  ud : Outport  Port=4
  ue : Outport  Port=5
  uf : Outport  Port=6
  wires:
  ua1/1 -> Subtract/1
  ua2/1 -> Subtract/2
  Subtract/1 -> ua/1
  ub1/1 -> Subtract1/1
  ub2/1 -> Subtract1/2
  Subtract1/1 -> ub/1
  uc1/1 -> Subtract2/1
  uc2/1 -> Subtract2/2
  Subtract2/1 -> uc/1
  ud1/1 -> Subtract3/1
  ud2/1 -> Subtract3/2
  Subtract3/1 -> ud/1
  ue1/1 -> Subtract4/1
  ue2/1 -> Subtract4/2
  Subtract4/1 -> ue/1
  uf1/1 -> Subtract5/1
  uf2/1 -> Subtract5/2
  Subtract5/1 -> uf/1

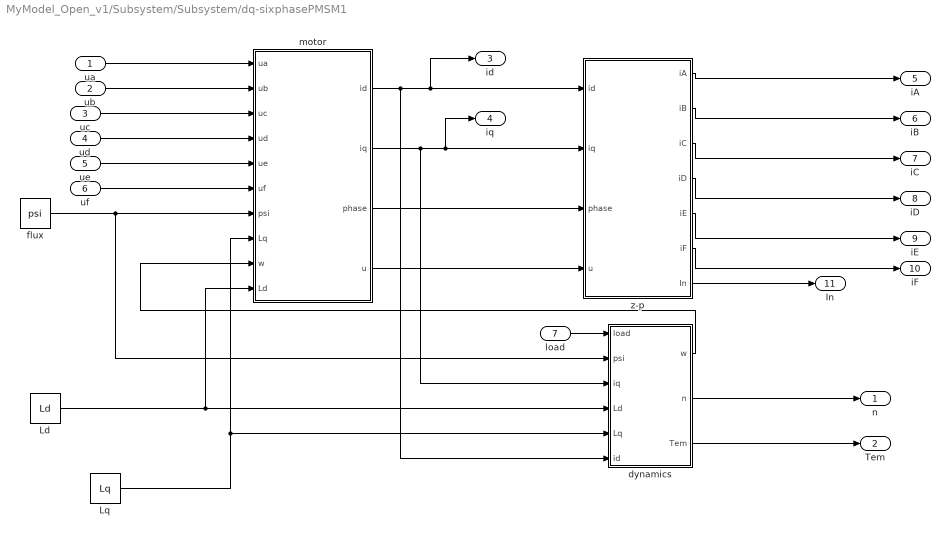
== system MyModel_Open_v1/Subsystem/Subsystem/dq-sixphasePMSM1 ==
  ua : Inport
  ub : Inport  Port=2
  uc : Inport  Port=3
  ud : Inport  Port=4
  ue : Inport  Port=5
  uf : Inport  Port=6
  load : Inport  Port=7
  Ld : Constant  Value=Ld
  Lq : Constant  Value=Lq
  dynamics : Subsystem
  flux : Constant  Value=psi
  motor : Subsystem
  z-p : Subsystem
  n : Outport
  Tem : Outport  Port=2
  id : Outport  Port=3
  iq : Outport  Port=4
  iA : Outport  Port=5
  iB : Outport  Port=6
  iC : Outport  Port=7
  iD : Outport  Port=8
  iE : Outport  Port=9
  iF : Outport  Port=10
  In : Outport  Port=11
  wires:
  Lq/1 -> motor/8(Lq), dynamics/5(Lq)
  Ld/1 -> dynamics/4(Ld), motor/10(Ld)
  ud/1 -> motor/4(ud)
  ua/1 -> motor/1(ua)
  ue/1 -> motor/5(ue)
  ub/1 -> motor/2(ub)
  uf/1 -> motor/6(uf)
  uc/1 -> motor/3(uc)
  dynamics/2(n) -> n/1
  load/1 -> dynamics/1(load)
  z-p/1(iA) -> iA/1
  motor/1(id) -> dynamics/6(id), z-p/1(id), id/1
  motor/2(iq) -> dynamics/3(iq), z-p/2(iq), iq/1
  motor/4(u) -> z-p/4(u)
  dynamics/1(w) -> motor/9(w)
  dynamics/3(Tem) -> Tem/1
  flux/1 -> dynamics/2(psi), motor/7(psi)
  z-p/2(iB) -> iB/1
  z-p/3(iC) -> iC/1
  z-p/4(iD) -> iD/1
  z-p/5(iE) -> iE/1
  z-p/6(iF) -> iF/1
  motor/3(phase) -> z-p/3(phase)
  z-p/7(In) -> In/1

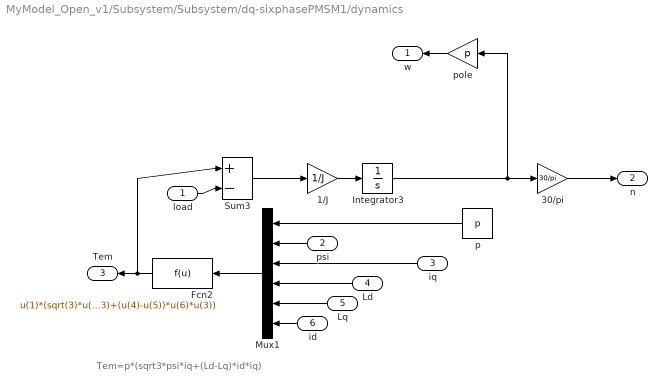
== system MyModel_Open_v1/Subsystem/Subsystem/dq-sixphasePMSM1/dynamics ==
  note: Tem=p*(sqrt3*psi*iq+(Ld-Lq)*id*iq)
  load : Inport
  psi : Inport  Port=2
  iq : Inport  Port=3
  Ld : Inport  Port=4
  Lq : Inport  Port=5
  id : Inport  Port=6
  1/J : Gain  Gain=1/J  SaturateOnIntegerOverflow=on  OutDataTypeStr=Inherit: Same as input  ParamDataTypeStr=Inherit: Same as input
  30/pi : Gain  Gain=30/pi  SaturateOnIntegerOverflow=on  OutDataTypeStr=Inherit: Same as input  ParamDataTypeStr=Inherit: Same as input
  Fcn2 : Fcn  Expr=u(1)*(sqrt(3)*u(2)*u(3)+(u(4)-u(5))*u(6)*u(3))
  Integrator3 : Integrator
  Mux1 : Mux  Inputs=6
  Sum3 : Sum  Inputs=|+-  SaturateOnIntegerOverflow=on
  p : Constant  Value=p
  pole : Gain  Gain=p  SaturateOnIntegerOverflow=on  OutDataTypeStr=Inherit: Same as input  ParamDataTypeStr=Inherit: Same as input
  w : Outport
  n : Outport  Port=2
  Tem : Outport  Port=3
  wires:
  p/1 -> Mux1/1
  Mux1/1 -> Fcn2/1
  Fcn2/1 -> Sum3/1, Tem/1
  Sum3/1 -> 1/J/1
  1/J/1 -> Integrator3/1
  Integrator3/1 -> 30/pi/1, pole/1
  psi/1 -> Mux1/2
  Ld/1 -> Mux1/4
  Lq/1 -> Mux1/5
  pole/1 -> w/1
  30/pi/1 -> n/1
  load/1 -> Sum3/2
  iq/1 -> Mux1/3
  id/1 -> Mux1/6

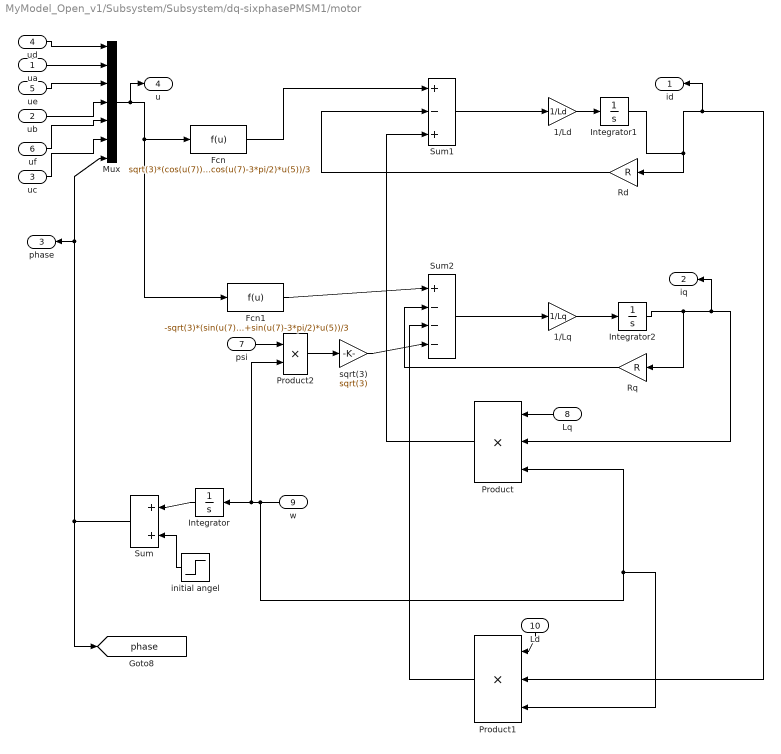
== system MyModel_Open_v1/Subsystem/Subsystem/dq-sixphasePMSM1/motor ==
  ua : Inport
  ub : Inport  Port=2
  uc : Inport  Port=3
  ud : Inport  Port=4
  ue : Inport  Port=5
  uf : Inport  Port=6
  psi : Inport  Port=7
  Lq : Inport  Port=8
  w : Inport  Port=9
  Ld : Inport  Port=10
  1/Ld : Gain  Gain=1/Ld  SaturateOnIntegerOverflow=on  OutDataTypeStr=Inherit: Same as input  ParamDataTypeStr=Inherit: Same as input
  1/Lq : Gain  Gain=1/Lq  SaturateOnIntegerOverflow=on  OutDataTypeStr=Inherit: Same as input  ParamDataTypeStr=Inherit: Same as input
  Fcn : Fcn  Expr=sqrt(3)*(cos(u(7))*u(2)+cos(u(7)-pi/6)*u(4)+cos(u(7)-2*pi/3)*u(6)+cos(u(7)-5*pi/6)*u(1)+cos(u(7)-4*pi/3)*u(3)+cos(u(7)-3*pi/2)*u(5))/3
  Fcn1 : Fcn  Expr=-sqrt(3)*(sin(u(7))*u(2)+sin(u(7)-pi/6)*u(4)+sin(u(7)-2*pi/3)*u(6)+sin(u(7)-5*pi/6)*u(1)+sin(u(7)-4*pi/3)*u(3)+sin(u(7)-3*pi/2)*u(5))/3
  Integrator : Integrator
  Integrator1 : Integrator
  Integrator2 : Integrator
  Mux : Mux  Inputs=7
  Product : Product  Inputs=3  SaturateOnIntegerOverflow=on  OutDataTypeStr=Inherit: Same as first input
  Product1 : Product  Inputs=3  SaturateOnIntegerOverflow=on  OutDataTypeStr=Inherit: Same as first input
  Product2 : Product  SaturateOnIntegerOverflow=on  OutDataTypeStr=Inherit: Same as first input
  Rd : Gain  Gain=R  SaturateOnIntegerOverflow=on  OutDataTypeStr=Inherit: Same as input  ParamDataTypeStr=Inherit: Same as input
  Rq : Gain  Gain=R  SaturateOnIntegerOverflow=on  OutDataTypeStr=Inherit: Same as input  ParamDataTypeStr=Inherit: Same as input
  Sum : Sum  Inputs=|++  SaturateOnIntegerOverflow=on
  Sum1 : Sum  Inputs=|+-+  SaturateOnIntegerOverflow=on
  Sum2 : Sum  Inputs=|+---  SaturateOnIntegerOverflow=on
  initial angel : Step  Time=0  After=13*pi/9  SampleTime=0
  sqrt(3) : Gain  Gain=sqrt(3)  SaturateOnIntegerOverflow=on  OutDataTypeStr=Inherit: Same as input  ParamDataTypeStr=Inherit: Same as input
  id : Outport
  iq : Outport  Port=2
  phase : Outport  Port=3
  u : Outport  Port=4
  tag scope: phase=global
  wires:
  Sum/1 -> Mux/7, phase/1, [phase]
  Integrator/1 -> Sum/1
  initial angel/1 -> Sum/2
  w/1 -> Product2/2, Integrator/1, Product1/3, Product/3
  Mux/1 -> Fcn/1, Fcn1/1, u/1
  Fcn/1 -> Sum1/1
  Sum1/1 -> 1/Ld/1
  1/Ld/1 -> Integrator1/1
  Integrator1/1 -> Rd/1, id/1, Product1/2
  Rd/1 -> Sum1/2
  Fcn1/1 -> Sum2/1
  Sum2/1 -> 1/Lq/1
  1/Lq/1 -> Integrator2/1
  Integrator2/1 -> Rq/1, iq/1, Product/2
  Rq/1 -> Sum2/2
  Product/1 -> Sum1/3
  Product1/1 -> Sum2/3
  Product2/1 -> sqrt(3)/1
  psi/1 -> Product2/1
  Lq/1 -> Product/1
  Ld/1 -> Product1/1
  ud/1 -> Mux/1
  ua/1 -> Mux/2
  ue/1 -> Mux/3
  ub/1 -> Mux/4
  uf/1 -> Mux/5
  uc/1 -> Mux/6
  sqrt(3)/1 -> Sum2/4

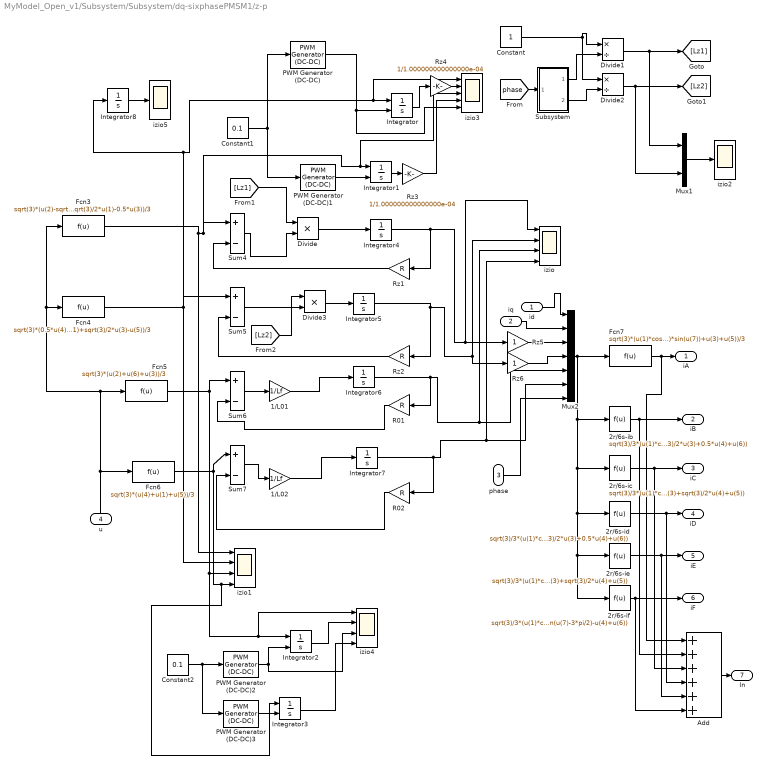
== system MyModel_Open_v1/Subsystem/Subsystem/dq-sixphasePMSM1/z-p ==
  id : Inport
  iq : Inport  Port=2
  phase : Inport  Port=3
  u : Inport  Port=4
  1/L01 : Gain  Gain=1/Lf  SaturateOnIntegerOverflow=on  OutDataTypeStr=Inherit: Same as input  ParamDataTypeStr=Inherit: Same as input
  1/L02 : Gain  Gain=1/Lf  SaturateOnIntegerOverflow=on  OutDataTypeStr=Inherit: Same as input  ParamDataTypeStr=Inherit: Same as input
  2r/6s-ib : Fcn  Expr=sqrt(3)/3*(u(1)*cos(u(7)-pi/6)-u(2)*sin(u(7)-pi/6)-sqrt(3)/2*u(3)+0.5*u(4)+u(6))
  2r/6s-ic : Fcn  Expr=sqrt(3)/3*(u(1)*cos(u(7)-2*pi/3)-u(2)*sin(u(7)-2*pi/3)-0.5*u(3)+sqrt(3)/2*u(4)+u(5))
  2r/6s-id : Fcn  Expr=sqrt(3)/3*(u(1)*cos(u(7)-5*pi/6)-u(2)*sin(u(7)-5*pi/6)+sqrt(3)/2*u(3)+0.5*u(4)+u(6))
  2r/6s-ie : Fcn  Expr=sqrt(3)/3*(u(1)*cos(u(7)-4*pi/3)-u(2)*sin(u(7)-4*pi/3)-0.5*u(3)+sqrt(3)/2*u(4)+u(5))
  2r/6s-if : Fcn  Expr=sqrt(3)/3*(u(1)*cos(u(7)-3*pi/2)-u(2)*sin(u(7)-3*pi/2)-u(4)+u(6))
  Add : Sum  Inputs=++++++
  Constant : Constant
  Constant1 : Constant  Value=0.1
  Constant2 : Constant  Value=0.1
  Divide : Product  Inputs=**
  Divide1 : Product  Inputs=*/
  Divide2 : Product  Inputs=*/
  Divide3 : Product  Inputs=**
  Fcn3 : Fcn  Expr=sqrt(3)*(u(2)-sqrt(3)/2*u(4)-0.5*u(6)+sqrt(3)/2*u(1)-0.5*u(3))/3
  Fcn4 : Fcn  Expr=sqrt(3)*(0.5*u(4)-sqrt(3)/2*u(6)+0.5*u(1)+sqrt(3)/2*u(3)-u(5))/3
  Fcn5 : Fcn  Expr=sqrt(3)*(u(2)+u(6)+u(3))/3
  Fcn6 : Fcn  Expr=sqrt(3)*(u(4)+u(1)+u(5))/3
  Fcn7 : Fcn  Expr=sqrt(3)*(u(1)*cos(u(7))-u(2)*sin(u(7))+u(3)+u(5))/3
  Integrator{,1..3} (4 alike) : Integrator  ExternalReset=rising
  Integrator{4..8} (5 alike) : Integrator
  Mux1 : Mux  Inputs=2
  Mux2 : Mux  Inputs=7
  PWM Generator (DC-DC){,1..3} (4 alike) : powerlib_meascontrol/Pulse & Signal Generators/PWM Generator (DC-DC)  Fsw=1/1.000000000000000e-04  Ts=0
  R01 : Gain  Gain=R  SaturateOnIntegerOverflow=on  OutDataTypeStr=Inherit: Same as input  ParamDataTypeStr=Inherit: Same as input
  R02 : Gain  Gain=R  SaturateOnIntegerOverflow=on  OutDataTypeStr=Inherit: Same as input  ParamDataTypeStr=Inherit: Same as input
  Rz1 : Gain  Gain=R  SaturateOnIntegerOverflow=on  OutDataTypeStr=Inherit: Same as input  ParamDataTypeStr=Inherit: Same as input
  Rz2 : Gain  Gain=R  SaturateOnIntegerOverflow=on  OutDataTypeStr=Inherit: Same as input  ParamDataTypeStr=Inherit: Same as input
  Rz3 : Gain  Gain=1/1.000000000000000e-04  SaturateOnIntegerOverflow=on  OutDataTypeStr=Inherit: Same as input  ParamDataTypeStr=Inherit: Same as input
  Rz4 : Gain  Gain=1/1.000000000000000e-04  SaturateOnIntegerOverflow=on  OutDataTypeStr=Inherit: Same as input  ParamDataTypeStr=Inherit: Same as input
  Rz5 : Gain  SaturateOnIntegerOverflow=on  OutDataTypeStr=Inherit: Same as input  ParamDataTypeStr=Inherit: Same as input
  Rz6 : Gain  SaturateOnIntegerOverflow=on  OutDataTypeStr=Inherit: Same as input  ParamDataTypeStr=Inherit: Same as input
  Subsystem : Subsystem
  Sum{4..7} (4 alike) : Sum  Inputs=|+-  SaturateOnIntegerOverflow=on
  izio : Scope  NumInputPorts=4
  izio1 : Scope  NumInputPorts=4
  izio2 : Scope
  izio3 : Scope  NumInputPorts=5
  izio4 : Scope  NumInputPorts=4
  izio5 : Scope
  iA : Outport
  iB : Outport  Port=2
  iC : Outport  Port=3
  iD : Outport  Port=4
  iE : Outport  Port=5
  iF : Outport  Port=6
  In : Outport  Port=7
  wires:
  Mux2/1 -> Fcn7/1, 2r/6s-ic/1, 2r/6s-id/1, 2r/6s-ie/1, 2r/6s-if/1, 2r/6s-ib/1
  R02/1 -> Sum7/2
  R01/1 -> Sum6/2
  Rz2/1 -> Sum5/2
  Rz1/1 -> Sum4/2
  Integrator7/1 -> R02/1, Mux2/6, izio/4
  1/L02/1 -> Integrator7/1
  Sum7/1 -> 1/L02/1
  Integrator6/1 -> R01/1, Mux2/5, izio/3
  1/L01/1 -> Integrator6/1
  Sum6/1 -> 1/L01/1
  id/1 -> Mux2/1
  iq/1 -> Mux2/2
  u/1 -> Fcn4/1, Fcn3/1, Fcn5/1, Fcn6/1
  phase/1 -> Mux2/7
  Fcn7/1 -> Add/1, iA/1
  2r/6s-ib/1 -> Add/2, iB/1
  2r/6s-id/1 -> Add/4, iD/1
  2r/6s-ie/1 -> Add/5, iE/1
  2r/6s-if/1 -> Add/6, iF/1
  [phase] -> Subsystem/1(Phase)
  Subsystem/1(Lz1) -> Divide1/2
  Divide1/1 -> Mux1/1, [Lz1]
  Constant/1 -> Divide1/1, Divide2/1
  Subsystem/2(Lz2) -> Divide2/2
  Divide2/1 -> Mux1/2, [Lz2]
  Mux1/1 -> izio2/1
  Sum4/1 -> Divide/2
  [Lz1] -> Divide/1
  Divide/1 -> Integrator4/1
  Divide3/1 -> Integrator5/1
  Sum5/1 -> Divide3/2
  [Lz2] -> Divide3/1
  Constant1/1 -> PWM Generator (DC-DC)/1, PWM Generator (DC-DC)1/1
  PWM Generator (DC-DC)/1 -> izio3/5, Integrator/2
  PWM Generator (DC-DC)1/1 -> Integrator1/2
  Fcn6/1 -> Sum7/1, Integrator3/1, izio1/4
  Fcn5/1 -> Sum6/1, izio4/1, Integrator2/1, izio1/3
  Constant2/1 -> PWM Generator (DC-DC)3/1, PWM Generator (DC-DC)2/1
  PWM Generator (DC-DC)2/1 -> Integrator2/2, izio4/3
  Integrator2/1 -> izio4/2
  PWM Generator (DC-DC)3/1 -> Integrator3/2
  Integrator3/1 -> izio4/4
  Integrator1/1 -> Rz3/1
  Rz3/1 -> izio3/4
  Integrator5/1 -> Rz2/1, Rz6/1, izio/2
  Rz4/1 -> izio3/2
  Integrator/1 -> Rz4/1
  Integrator4/1 -> Rz1/1, Rz5/1, izio/1
  Rz5/1 -> Mux2/3
  Rz6/1 -> Mux2/4
  Integrator8/1 -> izio5/1
  Fcn3/1 -> izio1/1, izio3/3, Integrator1/1, Sum4/1
  Fcn4/1 -> Sum5/1, izio3/1, Integrator/1, Integrator8/1, izio1/2
  Add/1 -> In/1
  2r/6s-ic/1 -> Add/3, iC/1

== system MyModel_Open_v1/Subsystem/Subsystem/dq-sixphasePMSM1/z-p/Subsystem ==
  Phase : Inport
  La0 : Constant  Value=-0.00139e-3
  La1 : Constant  Value=1.5201e-3
  La2 : Constant  Value=0.54985e-3
  Ldq_dmm1 : Scope  NumInputPorts=6
  Lg0 : Constant  Value=-0.0000798e-3
  Lg1 : Constant  Value=-0.000032e-3
  Lg2 : Constant  Value=-0.000052e-3
  "Manually Calculated Results " : MATLAB Function  TreatAsAtomicUnit=on
  Lz1 : Outport
  Lz2 : Outport  Port=2
  wires:
  "Manually Calculated Results "/3(Lz1) -> Lz1/1, Ldq_dmm1/3
  Lg2/1 -> "Manually Calculated Results "/6(Lg2)
  Lg1/1 -> "Manually Calculated Results "/5(Lg1)
  "Manually Calculated Results "/2(Lq) -> Ldq_dmm1/2
  Lg0/1 -> "Manually Calculated Results "/3(Lg0)
  "Manually Calculated Results "/4(Lz2) -> Lz2/1, Ldq_dmm1/4
  "Manually Calculated Results "/6(Lo2) -> Ldq_dmm1/6
  "Manually Calculated Results "/1(Ld) -> Ldq_dmm1/1
  "Manually Calculated Results "/5(Lo1) -> Ldq_dmm1/5
  La0/1 -> "Manually Calculated Results "/1(La0)
  La1/1 -> "Manually Calculated Results "/2(La1)
  La2/1 -> "Manually Calculated Results "/4(La2)
  Phase/1 -> "Manually Calculated Results "/7(RP)

== matlab function MyModel_Open_v1/Subsystem/Subsystem/dq-sixphasePMSM1/z-p/Subsystem/Manually Calculated Results  ==
  data: La0 input; Ld output; La1 input; Lg0 input; La2 input; Lg1 input; Lg2 input; RP input; Lq output; Lz1 output; Lz2 output; Lo1 output; Lo2 output
function [Ld,Lq,Lz1,Lz2,Lo1,Lo2] = fcn(La0,La1,Lg0,La2,Lg1,Lg2,RP)
%#codegen
Ld=3*La0+La1+sqrt(3)*La2+(1/2*Lg0+Lg1+Lg2);
Lq=3*La0+sqrt(3)*La2+La1-(1/2*Lg0+Lg1+Lg2);
Lz1=La1+cos(2*RP)*(1/2*Lg0-Lg1+Lg2)-sqrt(3)*La2;
Lz2=La1-cos(2*RP)*(1/2*Lg0-Lg1+Lg2)-sqrt(3)*La2;
Lo1=La1;
Lo2=La1;

== matlab function MyModel_Open_v1/Subsystem/Embedded MATLAB Function ==
  data: uo output; uab input; ua output; ubc input; ucd input; ude input; uef input; ub output; uc output; ud output; ue output; uf output
function [uo,ua,ub,uc,ud,ue,uf] = fcn(uab,ubc,ucd,ude,uef)

%#codegen
uxx = [uab,ubc,ucd,ude,uef,0,0]';
T = [0 1 -1 0 0 0 0;
     0 0 1 -1 0 0 0;
     1 0 0 1 -1 0 0;
     0 0 0 0 1 -1 0;
     0 0 0 0 0 1 -1;
     0 1 1 1 0 0 0;
     0 0 0 0 1 1 1];
I = T \ uxx;
uo = I(1);
ua = I(2);
ub = I(3);
uc = I(4);
ud = I(5);
ue = I(6);
uf = I(7);

== matlab function MyModel_Open_v1/Subsystem/Embedded MATLAB Function1 ==
  data: uo output; uab input; ua output; ubc input; ucd input; ude input; uef input; ub output; uc output; ud output; ue output; uf output
function [uo,ua,ub,uc,ud,ue,uf] = fcn(uab,ubc,ucd,ude,uef)

%#codegen
uxx = [uab,ubc,ucd,ude,uef,0,0]';
T = [0 1 -1 0 0 0 0;
     0 0 1 -1 0 0 0;
     1 0 0 1 -1 0 0;
     0 0 0 0 1 -1 0;
     0 0 0 0 0 1 -1;
     0 1 1 1 0 0 0;
     0 0 0 0 1 1 1];
I = T \ uxx;
uo = I(1);
ua = I(2);
ub = I(3);
uc = I(4);
ud = I(5);
ue = I(6);
uf = I(7);

== matlab function MyModel_Open_v1/Subsystem/clark1 ==
  data: falpha output; fa input; fbeta output; fb input; fc input; fd input; fe input; fx output; fy output; fo1 output; fo2 output; ff input
function [falpha,fbeta,fx,fy,fo1,fo2] = clark(fa,fb,fc,fd,fe,ff)

T=1/sqrt(3)*[1,  (-1/2),    (-1/2),       sqrt(3)/2,  -sqrt(3)/2,  0;
       0,  sqrt(3)/2, (-sqrt(3)/2), 1/2,        1/2,        -1;
       1,  (-1/2),    (-1/2),       -sqrt(3)/2, sqrt(3)/2,   0;
       0,  -sqrt(3)/2,sqrt(3)/2,    1/2,        1/2,        -1;
       1,  1,         1,            0,          0,           0;
       0,  0,         0,            1,          1,           1];
X=[fa;fb;fc;fd;fe;ff];
Y=T*X;
falpha=Y(1);
fbeta=Y(2);
fx=Y(3);
fy=Y(4);
fo1=Y(5);
fo2=Y(6);
end

== matlab function MyModel_Open_v1/SVPWM2/Embedded MATLAB Function2 ==
  data: N input; t1 output; Ualpha input; Ubeta input; Tpwm input; t2 output; t3 output; t4 output; t0 output; udc input; Ux input; Uy input; t1cp output; t2cp output; t3cp output; t4cp output
function [t1, t2, t3, t4, t0, t1cp, t2cp, t3cp, t4cp] = fcn(N, Ualpha, Ubeta, Tpwm, udc, Ux,Uy)

m=sqrt(3)/2+1/2*1i;

%等功率clarke反变换
ab44=1/sqrt(3)*udc*[1,m^4,m^8,m,m^5,m^9]*[1;0;0;1;0;0];
xy44=1/sqrt(3)*udc*[1,m^8,m^4,m^5,m,m^9]*[1;0;0;1;0;0];

ab64=1/sqrt(3)*udc*[1,m^4,m^8,m,m^5,m^9]*[1;1;0;1;0;0];
xy64=1/sqrt(3)*udc*[1,m^8,m^4,m^5,m,m^9]*[1;1;0;1;0;0];
        
ab66=1/sqrt(3)*udc*[1,m^4,m^8,m,m^5,m^9]*[1;1;0;1;1;0];
xy66=1/sqrt(3)*udc*[1,m^8,m^4,m^5,m,m^9]*[1;1;0;1;1;0];

ab26=1/sqrt(3)*udc*[1,m^4,m^8,m,m^5,m^9]*[0;1;0;1;1;0];
xy26=1/sqrt(3)*udc*[1,m^8,m^4,m^5,m,m^9]*[0;1;0;1;1;0];

ab22=1/sqrt(3)*udc*[1,m^4,m^8,m,m^5,m^9]*[0;1;0;0;1;0];
xy22=1/sqrt(3)*udc*[1,m^8,m^4,m^5,m,m^9]*[0;1;0;0;1;0];

ab32=1/sqrt(3)*udc*[1,m^4,m^8,m,m^5,m^9]*[0;1;1;0;1;0];
xy32=1/sqrt(3)*udc*[1,m^8,m^4,m^5,m,m^9]*[0;1;1;0;1;0];

ab33=1/sqrt(3)*udc*[1,m^4,m^8,m,m^5,m^9]*[0;1;1;0;1;1];
xy33=1/sqrt(3)*udc*[1,m^8,m^4,m^5,m,m^9]*[0;1;1;0;1;1];

ab13=1/sqrt(3)*udc*[1,m^4,m^8,m,m^5,m^9]*[0;0;1;0;1;1];
xy13=1/sqrt(3)*udc*[1,m^8,m^4,m^5,m,m^9]*[0;0;1;0;1;1];

ab11=1/sqrt(3)*udc*[1,m^4,m^8,m,m^5,m^9]*[0;0;1;0;0;1];
xy11=1/sqrt(3)*udc*[1,m^8,m^4,m^5,m,m^9]*[0;0;1;0;0;1];

ab51=1/sqrt(3)*udc*[1,m^4,m^8,m,m^5,m^9]*[1;0;1;0;0;1];
xy51=1/sqrt(3)*udc*[1,m^8,m^4,m^5,m,m^9]*[1;0;1;0;0;1];

ab55=1/sqrt(3)*udc*[1,m^4,m^8,m,m^5,m^9]*[1;0;1;1;0;1];
xy55=1/sqrt(3)*udc*[1,m^8,m^4,m^5,m,m^9]*[1;0;1;1;0;1];

ab45=1/sqrt(3)*udc*[1,m^4,m^8,m,m^5,m^9]*[1;0;0;1;0;1];
xy45=1/sqrt(3)*udc*[1,m^8,m^4,m^5,m,m^9]*[1;0;0;1;0;1];

switch N
    case 1
        X=[real(ab55),real(ab45),real(ab44),real(ab64);
           imag(ab55),imag(ab45),imag(ab44),imag(ab64);
           real(xy55),real(xy45),real(xy44),real(xy64);
           imag(xy55),imag(xy45),imag(xy44),imag(xy64)];

    case 2
        X=[real(ab45),real(ab44),real(ab64),real(ab66);
           imag(ab45),imag(ab44),imag(ab64),imag(ab66);
           real(xy45),real(xy44),real(xy64),real(xy66);
           imag(xy45),imag(xy44),imag(xy64),imag(xy66)];

    case 3
        X=[real(ab44),real(ab64),real(ab66),real(ab26);
           imag(ab44),imag(ab64),imag(ab66),imag(ab26);
           real(xy44),real(xy64),real(xy66),real(xy26);
           imag(xy44),imag(xy64),imag(xy66),imag(xy26)];

    case 4
        X=[real(ab64),real(ab66),real(ab26),real(ab22);
           imag(ab64),imag(ab66),imag(ab26),imag(ab22);
           real(xy64),real(xy66),real(xy26),real(xy22);
           imag(xy64),imag(xy66),imag(xy26),imag(xy22)];

    case 5
        X=[real(ab66),real(ab26),real(ab22),real(ab32);
           imag(ab66),imag(ab26),imag(ab22),imag(ab32);
           real(xy66),real(xy26),real(xy22),real(xy32);
           imag(xy66),imag(xy26),imag(xy22),imag(xy32)];

    case 6
        X=[real(ab26),real(ab22),real(ab32),real(ab33);
           imag(ab26),imag(ab22),imag(ab32),imag(ab33);
           real(xy26),real(xy22),real(xy32),real(xy33);
           imag(xy26),imag(xy22),imag(xy32),imag(xy33)];

    case 7
        X=[real(ab22),real(ab32),real(ab33),real(ab13);
           imag(ab22),imag(ab32),imag(ab33),imag(ab13);
           real(xy22),real(xy32),real(xy33),real(xy13);
           imag(xy22),imag(xy32),imag(xy33),imag(xy13)];

    case 8
        X=[real(ab32),real(ab33),real(ab13),real(ab11);
           imag(ab32),imag(ab33),imag(ab13),imag(ab11);
           real(xy32),real(xy33),real(xy13),real(xy11);
           imag(xy32),imag(xy33),imag(xy13),imag(xy11)];

    case 9
        X=[real(ab33),real(ab13),real(ab11),real(ab51);
           imag(ab33),imag(ab13),imag(ab11),imag(ab51);
           real(xy33),real(xy13),real(xy11),real(xy51);
           imag(xy33),imag(xy13),imag(xy11),imag(xy51)];

    case 10
        X=[real(ab13),real(ab11),real(ab51),real(ab55);
           imag(ab13),imag(ab11),imag(ab51),imag(ab55);
           real(xy13),real(xy11),real(xy51),real(xy55);
           imag(xy13),imag(xy11),imag(xy51),imag(xy55)];

    case 11
        X=[real(ab11),real(ab51),real(ab55),real(ab45);
           imag(ab11),imag(ab51),imag(ab55),imag(ab45);
           real(xy11),real(xy51),real(xy55),real(xy45);
           imag(xy11),imag(xy51),imag(xy55),imag(xy45)];

    case 12
        X=[real(ab51),real(ab55),real(ab45),real(ab44);
           imag(ab51),imag(ab55),imag(ab45),imag(ab44);
           real(xy51),real(xy55),real(xy45),real(xy44);
           imag(xy51),imag(xy55),imag(xy45),imag(xy44)];

    otherwise
        X=[0,0,0,0;
           0,0,0,0;
           0,0,0,0;
           0,0,0,0];

end
Y=[Ualpha;Ubeta;Ux;Uy]*Tpwm;
T = X \ Y;

% t1=T(1);
% if t1<15e-6
%     t1=15e-6;
% end
% t2=T(2);
% if t2<15e-6
%     t2=15e-6;
% end
% t3=T(3);
% if t3<1e-6
%     t3=1e-6;
% end
% t4=T(4);
% if t4<1e-6
%     t4=1e-6;
% end

% T1=T(1);
% T2=T(2);
% T3=T(3);
% T4=T(4);
t1cp = 0;
t2cp = 0;
t3cp = 0;
t4cp = 0;
if T(1) >= 0
    t1 = T(1);
else
    t1 = 0;
    t1cp = -T(1);
end
if T(2) >= 0
    t2 = T(2);
else
    t2 = 0;
    t2cp = -T(2);
end
if T(3) >= 0
    t3 = T(3);
else
    t3 = 0;
    t3cp = -T(3);
end
if T(4) >= 0
    t4 = T(4);
else
    t4 = 0;
    t4cp = -T(4);
end

Tsum=t1+t2+t3+t4;
if Tsum>Tpwm
    t1=t1*Tpwm/Tsum;
    t2=t2*Tpwm/Tsum;
    t3=t3*Tpwm/Tsum;
    t4=t4*Tpwm/Tsum;
end
t0=Tpwm-t1-t2-t3-t4;
end

== matlab function MyModel_Open_v1/SVPWM2/Embedded MATLAB Function6 ==
  data: N output; ualfa input; ubeta input; TH output
function [N,TH] = fcn(ualfa,ubeta)

%#xsxx
[TH,~] = cart2pol(ualfa,ubeta);
if TH<0
    TH=TH+2*pi;
end
N=floor((TH+pi/12)/(pi/6))+1;
if N==13
    N=1;
end

== matlab function MyModel_Open_v1/SVPWM2/rest of others ==
  data: N input; T1 input; T2 input; T3 input; T4 input; T0 input; a1 output; a2 output; b1 output; b2 output; c1 output; c2 output; d1 output; d2 output; e1 output; e2 output; f1 output; f2 output; t1cp input; t2cp input; t3cp input; t4cp input
function [a1,a2,b1,b2,c1,c2,d1,d2,e1,e2,f1,f2] = fcn(N,T1,T2,T3,T4,T0,t1cp,t2cp,t3cp,t4cp)

%#xsxx
Ta=T0/4;
Tb=Ta+T2;
Tc=Tb+T1;
Td=Tc+T0/2;
Te=Td+T4;
Tf=Te+T3;

Ta1=T0/4;
Tb1=Ta1+T1;
Tc1=Tb1+T2;
Td1=Tc1+T0/2;
Te1=Td1+T3;
Tf1=Te1+T4;

%a1:phase A CMPA
%a2:phase A CMPB

a1 = 0;
a2 = 0;
b1 = 0;
b2 = 0;
c1 = 0;
c2 = 0;
d1 = 0;
d2 = 0;
e1 = 0;
e2 = 0;
f1 = 0;
f2 = 0;

if N==1
    a1=Ta;%TIme of "00" voltage vector 
    a2=Tf;%TIme of "48" voltage vector 
    d1=Ta;
    d2=Tf;
    b1=Tc;%TIme of "51" voltage vector 
    b2=Te + t1cp + t2cp + t3cp;%TIme of "56" voltage vector 
    e1=Tc;
    e2=Td + t1cp +t2cp +t3cp + t4cp;
    c1=Tb;%TIme of "49" voltage vector 
    c2=Td + t2cp + t3cp + t4cp;%TIme of "63" voltage vector 
    f1=Ta;
    f2=Td + t3cp + t4cp;
elseif N==2
    a1=Ta;
    a2=Tf;
    d1=Ta;
    d2=Tf;
    b1=Tc;
    b2=Tf + t1cp + t2cp;
    e1=Tc;
    e2=Te + t1cp + t2cp + t3cp;
    c1=Tc;
    c2=Td + t1cp + t2cp + t3cp + t4cp;
    f1=Tb;
    f2=Td + t2cp + t3cp + t4cp;
elseif N==3
    a1=Ta1;
    a2=Te1 + t4cp;
    d1=Ta1;
    d2=Tf1;
    b1=Tb1;
    b2=Tf1 + t1cp;
    e1=Tc1;
    e2=Tf1 + t1cp + t2cp;
    c1=Tc1;
    c2=Td1 + t1cp + t2cp + t3cp + t4cp;
    f1=Tc1;
    f2=Td1 + t1cp + t2cp + t3cp + t4cp;
elseif N==4
    a1=Ta1;
    a2=Td1 + t3cp + t4cp;
    d1=Ta1;
    d2=Te1 + t4cp;
    b1=Ta1;
    b2=Tf1;
    e1=Tb1;
    e2=Tf1 + t1cp;
    c1=Tc1;
    c2=Td1 + t1cp + t2cp + t3cp + t4cp;
    f1=Tc1;
    f2=Td1 + t1cp + t2cp + t3cp + t4cp;
elseif N==5
    a1=Tb;
    a2=Td + t2cp + t3cp + t4cp;
    d1=Ta;
    d2=Td + t3cp + t4cp;
    b1=Ta;
    b2=Tf;
    e1=Ta;
    e2=Tf;
    c1=Tc;
    c2=Te + t1cp + t2cp + t3cp;
    f1=Tc;
    f2=Td + t1cp + t2cp + t3cp + t4cp;
elseif N==6
    a1=Tc;
    a2=Td + t1cp + t2cp + t3cp + t4cp;
    d1=Tb;
    d2=Td + t2cp + t3cp + t4cp;
    b1=Ta;
    b2=Tf;
    e1=Ta;
    e2=Tf;
    c1=Tc;
    c2=Tf + t1cp + t2cp;
    f1=Tc;
    f2=Te + t1cp + t2cp + t3cp;
elseif N==7
    a1=Tc1;
    a2=Td1 + t1cp + t2cp + t3cp + t4cp;
    d1=Tc1;
    d2=Td1 + t1cp + t2cp + t3cp + t4cp;
    b1=Ta1;
    b2=Te1 + t4cp;
    e1=Ta1;
    e2=Tf1;
    c1=Tb1;
    c2=Tf1 + t1cp;
    f1=Tc1;
    f2=Tf1 + t1cp + t2cp;
elseif N==8
    a1=Tc1;
    a2=Td1 + t1cp + t2cp + t3cp + t4cp;
    d1=Tc1;
    d2=Td1 + t1cp + t2cp + t3cp + t4cp;
    b1=Ta1;
    b2=Td1 + t3cp + t4cp;
    e1=Ta1;
    e2=Te1 + t4cp;
    c1=Ta1;
    c2=Tf1;
    f1=Tb1;
    f2=Tf1 + t1cp;
elseif N==9
    a1=Tc;
    a2=Te + t1cp + t2cp + t3cp;
    d1=Tc;
    d2=Td + t1cp + t2cp + t3cp + t4cp;
    b1=Tb;
    b2=Td + t2cp + t3cp + t4cp;
    e1=Ta;
    e2=Td + t3cp + t4cp;
    c1=Ta;
    c2=Tf;
    f1=Ta;
    f2=Tf;
elseif N==10
    a1=Tc;
    a2=Tf + t1cp + t2cp;
    d1=Tc;
    d2=Te + t1cp + t2cp + t3cp;
    b1=Tc;
    b2=Td + t1cp + t2cp + t3cp + t4cp;
    e1=Tb;
    e2=Td + t2cp + t3cp + t4cp;
    c1=Ta;
    c2=Tf;
    f1=Ta;
    f2=Tf;
elseif N==11
    a1=Tb1;
    a2=Tf1 + t1cp;
    d1=Tc1;
    d2=Tf1 + t1cp + t2cp;
    b1=Tc1;
    b2=Td1 + t1cp + t2cp + t3cp + t4cp;
    e1=Tc1;
    e2=Td1 + t1cp + t2cp + t3cp + t4cp;
    c1=Ta1;
    c2=Te1 + t4cp;
    f1=Ta1;
    f2=Tf1;
elseif N==12
    a1=Ta1;
    a2=Tf1;
    d1=Tb1;
    d2=Tf1 + t1cp;
    b1=Tc1;
    b2=Td1 + t1cp + t2cp + t3cp + t4cp;
    e1=Tc1;
    e2=Td1 + t1cp + t2cp + t3cp + t4cp;
    c1=Ta1;
    c2=Td1 + t3cp + t4cp;
    f1=Ta1;
    f2=Te1 + t4cp;
end
